simulink model "C172S_PitchAttitudeHold_V2_Actuator"  (R2026a)
settings: Solver=ode4  StartTime=0  StopTime=60  FixedStep=0.001
InitFcn:
  | pa2Data = c172sLongitudinalData();
  | [~,pa2Plant] = c172sLongitudinalPlant(pa2Data);
  | pa2Controller = c172sPitchAttitudeControllerData();
  | pa2Actuator = c172sElevatorActuatorData();
  | A_pa2 = pa2Plant.A; B_pa2 = pa2Plant.B;
  | C_pa2 = pa2Plant.C; D_pa2 = pa2Plant.D;
  | Kp_pa2 = pa2Controller.Kp_radPerRad;
  | Ki_pa2_per_s = pa2Controller.Ki_radPerRadPerS;
  | Kq_pa2_s = pa2Actuator.integration.Kq_s;
  | tauCommand_pa2_s = pa2Controller.commandFilterTimeConstant_s;
  | tauActuator_pa2_s = pa2Actuator.dynamics.timeConstant_s;
  | Tt_pa2_s = pa2Actuator.antiWindup.trackingTimeConstant_s;
  | deltaELower_pa2_rad = pa2Actuator.authority.lowerLimit_rad;
  | deltaEUpper_pa2_rad = pa2Actuator.authority.upperLimit_rad;
  | deltaERate_pa2_radps = deg2rad(pa2Actuator.dynamics.rateLimit_degps);
  | if ~exist('thetaCommand_pa2_rad','var'), thetaCommand_pa2_rad = deg2rad(pa2Actuator.validation.commandStep_deg); end
  | if ~exist('antiWindupEnable_pa2','var'), antiWindupEnable_pa2 = 1.0; end
  | if ~exist('x0_pa2','var'), x0_pa2 = zeros(4,1); end
  | if ~exist('xi0_pa2','var'), xi0_pa2 = 0.0; end
  | if ~exist('deltaE0_pa2','var'), deltaE0_pa2 = 0.0; end
undefined symbols (not defined in the file or in its folder): antiWindupEnable_pa2, deltaE0_pa2, x0_pa2, xi0_pa2
settings Model: Creator=Shahi  LastModifiedBy=Shahi

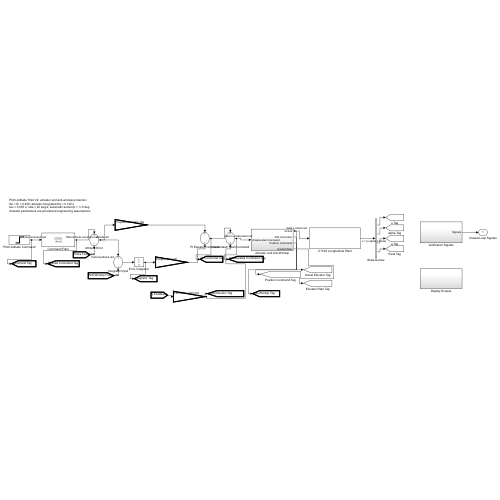
[thumbnail: Simulink's stored preview of the top-level diagram]
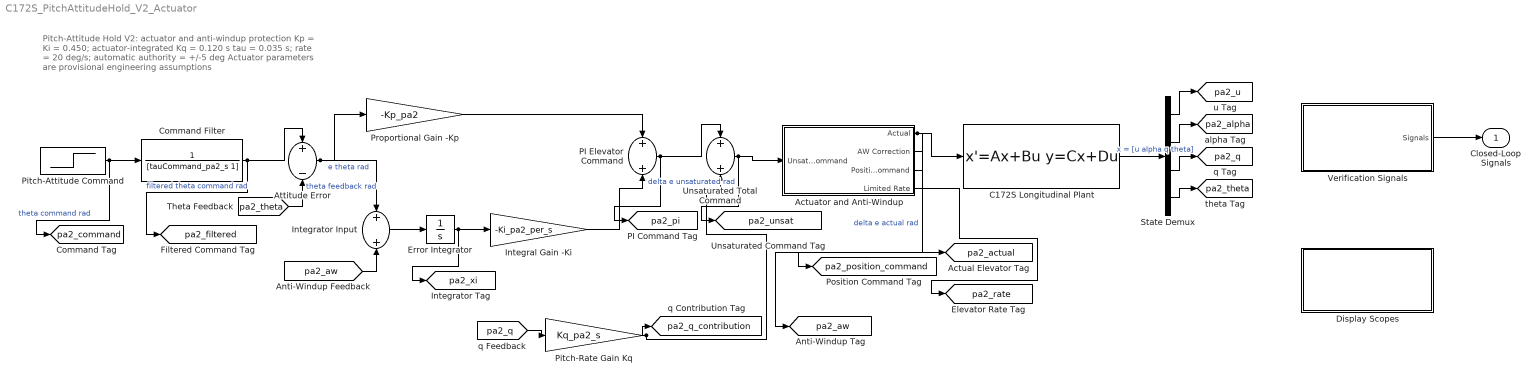
== system C172S_PitchAttitudeHold_V2_Actuator ==
  note: Pitch-Attitude Hold V2: actuator and anti-windup protection
      | Kp = Ki = 0.450; actuator-integrated Kq = 0.120 s
      | tau = 0.035 s; rate = 20 deg/s; automatic authority = +/-5 deg
      | Actuator parameters are provisional engineering assumptions
  Actuator and Anti-Windup : Subsystem
  Attitude Error : Sum  Inputs=+-
  C172S Longitudinal Plant : StateSpace  A=A_pa2  B=B_pa2  C=C_pa2  D=D_pa2  InitialCondition=x0_pa2
  Command Filter : TransferFcn  Numerator=1  Denominator=[tauCommand_pa2_s 1]
  Display Scopes : Subsystem
  Error Integrator : Integrator  InitialCondition=xi0_pa2
  Integral Gain -Ki : Gain  Gain=-Ki_pa2_per_s
  Integrator Input : Sum
  PI Elevator Command : Sum
  Pitch-Attitude Command : Step  Time=0  FinalValue=thetaCommand_pa2_rad  SampleTime=0
  Pitch-Rate Gain Kq : Gain  Gain=Kq_pa2_s
  Proportional Gain -Kp : Gain  Gain=-Kp_pa2
  State Demux : Demux
  Unsaturated Total Command : Sum
  Verification Signals : Subsystem
  Closed-Loop Signals : Outport
  tag scope: pa2_actual=global, pa2_alpha=global, pa2_aw=global, pa2_command=global, pa2_filtered=global, pa2_pi=global, pa2_position_command=global, pa2_q=global, pa2_q_contribution=global, pa2_rate=global, pa2_theta=global, pa2_u=global, pa2_unsat=global, pa2_xi=global
  wires:
  Verification Signals/1(Signals) -> Closed-Loop Signals/1
  Pitch-Attitude Command/1 -> Command Filter/1, [pa2_command]  "theta command rad"
  Command Filter/1 -> Attitude Error/1, [pa2_filtered]  "filtered theta command rad"
  [pa2_theta] -> Attitude Error/2  "theta feedback rad"
  Attitude Error/1 -> Proportional Gain -Kp/1, Integrator Input/1  "e theta rad"
  [pa2_aw] -> Integrator Input/2
  Integrator Input/1 -> Error Integrator/1
  Error Integrator/1 -> Integral Gain -Ki/1, [pa2_xi]
  Proportional Gain -Kp/1 -> PI Elevator Command/1
  Integral Gain -Ki/1 -> PI Elevator Command/2
  [pa2_q] -> Pitch-Rate Gain Kq/1
  PI Elevator Command/1 -> Unsaturated Total Command/1, [pa2_pi]
  Pitch-Rate Gain Kq/1 -> Unsaturated Total Command/2, [pa2_q_contribution]
  Unsaturated Total Command/1 -> Actuator and Anti-Windup/1(Unsaturated Command), [pa2_unsat]  "delta e unsaturated rad"
  Actuator and Anti-Windup/1(Actual) -> C172S Longitudinal Plant/1, [pa2_actual]  "delta e actual rad"
  C172S Longitudinal Plant/1 -> State Demux/1  "x = [u alpha q theta]"
  Actuator and Anti-Windup/2(AW Correction) -> [pa2_aw]
  Actuator and Anti-Windup/3(Position Command) -> [pa2_position_command]
  Actuator and Anti-Windup/4(Limited Rate) -> [pa2_rate]
  State Demux/1 -> [pa2_u]
  State Demux/2 -> [pa2_alpha]
  State Demux/3 -> [pa2_q]
  State Demux/4 -> [pa2_theta]

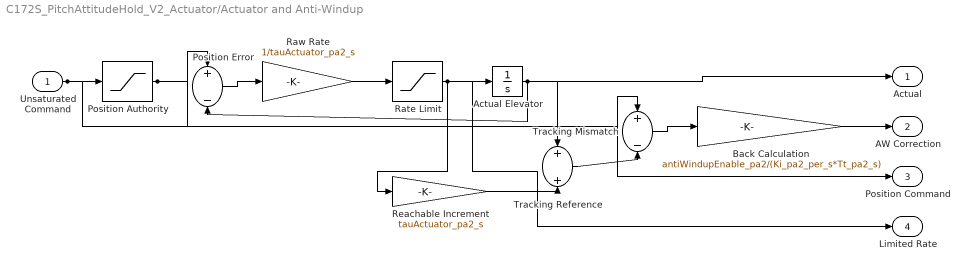
== system C172S_PitchAttitudeHold_V2_Actuator/Actuator and Anti-Windup ==
  Unsaturated Command : Inport
  Actual Elevator : Integrator  InitialCondition=deltaE0_pa2
  Back Calculation : Gain  Gain=antiWindupEnable_pa2/(Ki_pa2_per_s*Tt_pa2_s)
  Position Authority : Saturate  UpperLimit=deltaEUpper_pa2_rad  LowerLimit=deltaELower_pa2_rad
  Position Error : Sum  Inputs=+-
  Rate Limit : Saturate  UpperLimit=deltaERate_pa2_radps  LowerLimit=-deltaERate_pa2_radps
  Raw Rate : Gain  Gain=1/tauActuator_pa2_s
  Reachable Increment : Gain  Gain=tauActuator_pa2_s
  Tracking Mismatch : Sum  Inputs=+-
  Tracking Reference : Sum
  Actual : Outport
  AW Correction : Outport  Port=2
  Position Command : Outport  Port=3
  Limited Rate : Outport  Port=4
  wires:
  Unsaturated Command/1 -> Position Authority/1, Tracking Mismatch/1
  Position Authority/1 -> Position Error/1, Position Command/1
  Position Error/1 -> Raw Rate/1
  Raw Rate/1 -> Rate Limit/1
  Rate Limit/1 -> Actual Elevator/1, Reachable Increment/1, Limited Rate/1
  Actual Elevator/1 -> Position Error/2, Tracking Reference/1, Actual/1
  Reachable Increment/1 -> Tracking Reference/2
  Tracking Reference/1 -> Tracking Mismatch/2
  Tracking Mismatch/1 -> Back Calculation/1
  Back Calculation/1 -> AW Correction/1

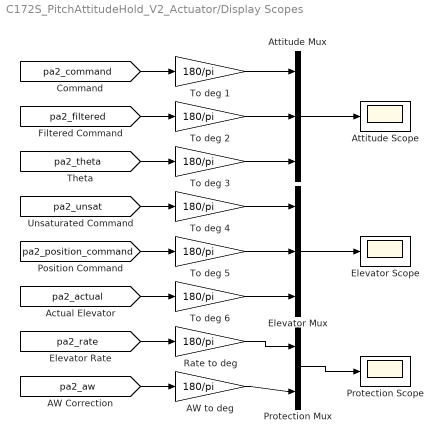
== system C172S_PitchAttitudeHold_V2_Actuator/Display Scopes ==
  AW to deg : Gain  Gain=180/pi
  Attitude Mux : Mux  Inputs=3
  Attitude Scope : Scope
  Elevator Mux : Mux  Inputs=3
  Elevator Scope : Scope
  Protection Mux : Mux  Inputs=2
  Protection Scope : Scope
  Rate to deg : Gain  Gain=180/pi
  To deg {1..6} (6 alike) : Gain  Gain=180/pi
  wires:
  [pa2_command] -> To deg 1/1
  [pa2_filtered] -> To deg 2/1
  [pa2_theta] -> To deg 3/1
  [pa2_unsat] -> To deg 4/1
  [pa2_position_command] -> To deg 5/1
  [pa2_actual] -> To deg 6/1
  To deg 1/1 -> Attitude Mux/1
  To deg 2/1 -> Attitude Mux/2
  To deg 3/1 -> Attitude Mux/3
  Attitude Mux/1 -> Attitude Scope/1
  To deg 4/1 -> Elevator Mux/1
  To deg 5/1 -> Elevator Mux/2
  To deg 6/1 -> Elevator Mux/3
  Elevator Mux/1 -> Elevator Scope/1
  [pa2_rate] -> Rate to deg/1
  [pa2_aw] -> AW to deg/1
  Rate to deg/1 -> Protection Mux/1
  AW to deg/1 -> Protection Mux/2
  Protection Mux/1 -> Protection Scope/1

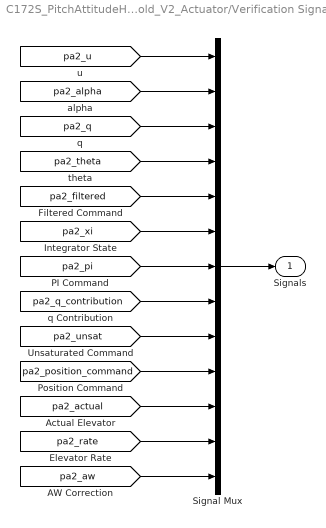
== system C172S_PitchAttitudeHold_V2_Actuator/Verification Signals ==
  Signal Mux : Mux  Inputs=13
  Signals : Outport
  wires:
  [pa2_u] -> Signal Mux/1
  [pa2_alpha] -> Signal Mux/2
  [pa2_q] -> Signal Mux/3
  [pa2_theta] -> Signal Mux/4
  [pa2_filtered] -> Signal Mux/5
  [pa2_xi] -> Signal Mux/6
  [pa2_pi] -> Signal Mux/7
  [pa2_q_contribution] -> Signal Mux/8
  [pa2_unsat] -> Signal Mux/9
  [pa2_position_command] -> Signal Mux/10
  [pa2_actual] -> Signal Mux/11
  [pa2_rate] -> Signal Mux/12
  [pa2_aw] -> Signal Mux/13
  Signal Mux/1 -> Signals/1
